simulink model "Filter"  (R2020b)
settings: Solver=VariableStepAuto  StartTime=0.0  StopTime=10.0  RelTol=1e-3
settings Model: Creator=MSI  LastModifiedBy=MSI

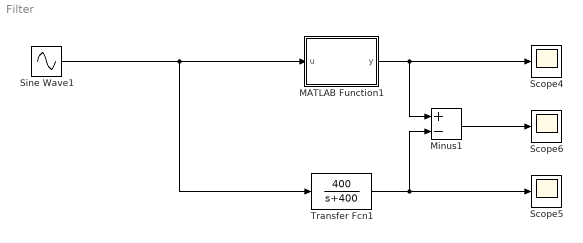
== system Filter ==
  MATLAB Function1 : MATLAB Function  TreatAsAtomicUnit=on
  Minus1 : Sum  Inputs=+-
  Scope4 : Scope
  Scope5 : Scope
  Scope6 : Scope
  Sine Wave1 : Sin  SampleTime=0  VectorParams1D=off
  Transfer Fcn1 : TransferFcn  Numerator=[400]  Denominator=[1 400]
  wires:
  Transfer Fcn1/1 -> Minus1/2, Scope5/1
  Sine Wave1/1 -> Transfer Fcn1/1, MATLAB Function1/1(u)
  Minus1/1 -> Scope6/1
  MATLAB Function1/1(y) -> Minus1/1, Scope4/1

== matlab function Filter/MATLAB Function1 ==
  settings: updateMethod=DISCRETE  sampleTime=1/500
  data: u input; y output
function y = Filter(u)

persistent Prev
persistent ept
persistent Temp
Tsample = 1/500;
nhat = 12;               % Number of samples taken/kept
P = 4/(Tsample*nhat)                 % Pole

% Initialize Temp
if isempty(Temp)
    Temp = 0;
end

% Initialize ept
if isempty(ept)
    ept = zeros(1, nhat);
    total = 0;
    for i = 1:nhat
        calc = P*exp(-P*i*Tsample);
        ept(i) = calc;
        total = total + calc;
    end
    scale = 1/(Tsample*total)
    ept = ept*scale*Tsample
end

% Initialize Prev
if isempty(Prev)
    Prev = zeros(1,nhat);
end

% Compute
Prev(1) = u
y = dot(ept, Prev)

% Take a step in time
for n = 1:(nhat - 1)
    Prev(nhat + 1 - n) = Prev(nhat - n);
end

Temp = u;
end
